simulink model "Level27"  (R2016a)
settings: Solver=VariableStepAuto  StartTime=0.0  StopTime=4/50  MaxStep=1e-6  MinStep=1e-7  RelTol=1e-3
libraries: simulink x26, powerlib x19
settings Model: Creator=satheeshwaran  LastModifiedBy=satheeshwaran

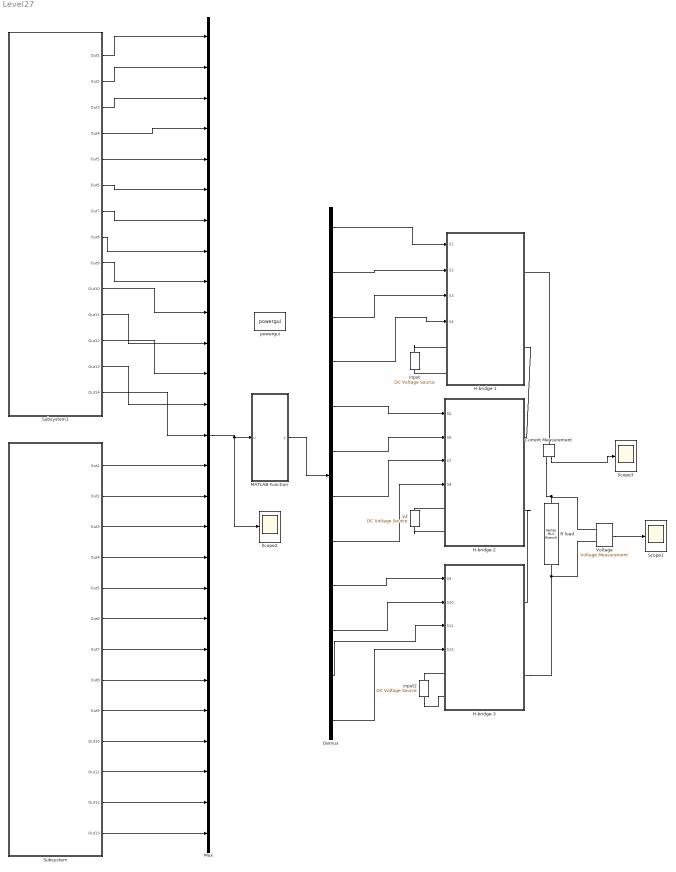
== system Level27 ==
  Current Measurement : powerlib/Measurements/Current Measurement  PhasorSimulation=off  OutputType=Complex  PSBequivalent=0
  Demux : Demux  Outputs=12
  H-bridge-1 : Subsystem
  H-bridge-2 : Subsystem
  H-bridge-3 : Subsystem
  MATLAB Function : MATLAB Function  TreatAsAtomicUnit=on
  Mux : Mux  Inputs=27
  R load : powerlib/Elements/Series RLC Branch  LConnTagsString=__new0  RConnTagsString=__new0  BranchType=R  Resistance=100  Inductance=1e-3  SetiL0=off  InitialCurrent=0  Capacitance=1e-6  Setx0=off  InitialVoltage=0  Measurements=None
  Scope1 : Scope
  Scope2 : Scope
  Scope3 : Scope
  Subsystem : Subsystem
  Subsystem1 : Subsystem
  Voltage : powerlib/Measurements/Voltage Measurement  PhasorSimulation=off  OutputType=Complex  PSBequivalent=0
  input : powerlib/Electrical Sources/DC Voltage Source  Amplitude=100  Measurements=None
  input2 : powerlib/Electrical Sources/DC Voltage Source  Amplitude=900  Measurements=None
  powergui : powerlib/powergui  Priority=1  SimulationMode=Continuous  SolverType=Tustin/Backward Euler (TBE)  SampleTime=50e-6  frequency=60  SPID=off  DisableSnubberDevices=off  DisableRonSwitches=off  DisableVfSwitches=off  SwTol=0  DisplayEquations=off  Interpol=off  ExternalGateDelay=off  methode=off  Ts=10  FunctionMessages=off  echomessages=off  HookPort=off  EnableUseOfTLC=off  x0status=blocks  frequencyindice=0  Pbase=100e6  ErrMax=1e-4  Iterations=50  UnitsV=kV  UnitsW=MW  buscounter=0  RestoreLinks=warning  ResistiveCurrentMeasurement=off  Frange=[0:2:500]  Ylog=off  Xlog=on  ShowGrid=off  save=off  variable=ZData  structure=vload  ZoomFFT=off  StartTime=0.04  cycles=1  DisplayStyle=1  fundamental=50  FreqAxis=off  MaxFrequency=20000  frequencyindicesteady=1  RmsSteady=1  display=off
  v2 : powerlib/Electrical Sources/DC Voltage Source  Amplitude=300  Measurements=None
  wires:
  Voltage/1 -> Scope1/1
  Demux/1 -> H-bridge-1/1(S1)
  Demux/2 -> H-bridge-1/2(S2)
  Demux/5 -> H-bridge-2/1(S5)
  Demux/6 -> H-bridge-2/2(S6)
  Demux/7 -> H-bridge-2/3(S7)
  Demux/9 -> H-bridge-3/1(S9)
  Demux/12 -> H-bridge-3/4(S12)
  Demux/11 -> H-bridge-3/3(S11)
  Demux/10 -> H-bridge-3/2(S10)
  Mux/1 -> Scope2/1, MATLAB Function/1(u)
  MATLAB Function/1(y) -> Demux/1
  Demux/3 -> H-bridge-1/3(S3)
  Demux/4 -> H-bridge-1/4(S4)
  Subsystem1/1(Out1) -> Mux/1
  Subsystem1/2(Out2) -> Mux/2
  Subsystem1/3(Out3) -> Mux/3
  Subsystem1/4(Out4) -> Mux/4
  Subsystem1/5(Out5) -> Mux/5
  Subsystem1/6(Out6) -> Mux/6
  Subsystem1/7(Out7) -> Mux/7
  Subsystem1/8(Out8) -> Mux/8
  Subsystem1/9(Out9) -> Mux/9
  Subsystem1/10(Out10) -> Mux/10
  Subsystem1/11(Out11) -> Mux/11
  Subsystem1/12(Out12) -> Mux/12
  Subsystem1/13(Out13) -> Mux/13
  Subsystem1/14(Out14) -> Mux/14
  Subsystem/1(Out1) -> Mux/15
  Subsystem/2(Out2) -> Mux/16
  Subsystem/3(Out3) -> Mux/17
  Subsystem/4(Out4) -> Mux/18
  Subsystem/5(Out5) -> Mux/19
  Subsystem/6(Out6) -> Mux/20
  Subsystem/7(Out7) -> Mux/21
  Subsystem/8(Out8) -> Mux/22
  Subsystem/9(Out9) -> Mux/23
  Subsystem/10(Out10) -> Mux/24
  Subsystem/11(Out11) -> Mux/25
  Subsystem/12(Out12) -> Mux/26
  Subsystem/13(Out13) -> Mux/27
  Demux/8 -> H-bridge-2/4(S8)
  Current Measurement/1 -> Scope3/1
  connections:
  Voltage/LConn2 -- H-bridge-3/RConn2 -- R load/RConn1
  input2/RConn1 -- H-bridge-3/LConn1
  input2/LConn1 -- H-bridge-3/LConn2
  H-bridge-2/RConn2 -- H-bridge-3/RConn1
  Voltage/LConn1 -- Current Measurement/RConn1 -- R load/LConn1
  H-bridge-1/RConn2 -- H-bridge-2/RConn1
  H-bridge-2/LConn1 -- v2/RConn1
  H-bridge-1/LConn2 -- input/LConn1
  v2/LConn1 -- H-bridge-2/LConn2
  input/RConn1 -- H-bridge-1/LConn1
  Current Measurement/LConn1 -- H-bridge-1/RConn1

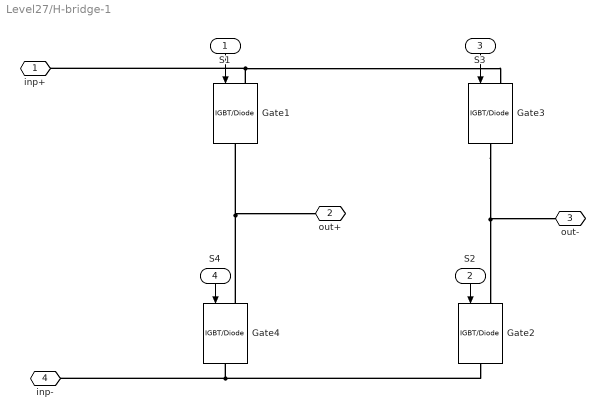
== system Level27/H-bridge-1 ==
  S1 : Inport
  S2 : Inport  Port=2
  S3 : Inport  Port=3
  S4 : Inport  Port=4
  Gate{1..4} (4 alike) : powerlib/Power Electronics/IGBT//Diode  Ron=1e-3  Rs=1e5  Cs=inf  Measurements=off
  inp+ : PMIOPort  Port=1  Side=Left
  out+ : PMIOPort  Port=2  Side=Right
  out- : PMIOPort  Port=3  Side=Right
  inp- : PMIOPort  Port=4  Side=Left
  wires:
  S1/1 -> Gate1/1
  S4/1 -> Gate4/1
  S2/1 -> Gate2/1
  S3/1 -> Gate3/1
  connections:
  Gate2/RConn1 -- inp-/RConn1 -- Gate4/RConn1
  Gate3/RConn1 -- out-/RConn1 -- Gate2/LConn1
  Gate4/LConn1 -- out+/RConn1 -- Gate1/RConn1
  Gate1/LConn1 -- inp+/RConn1 -- Gate3/LConn1

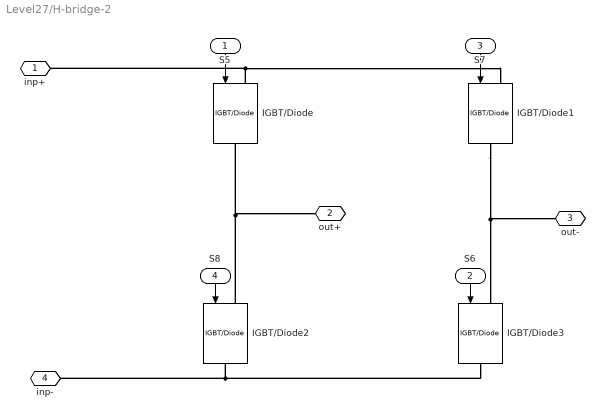
== system Level27/H-bridge-2 ==
  S5 : Inport
  S6 : Inport  Port=2
  S7 : Inport  Port=3
  S8 : Inport  Port=4
  IGBT/Diode{,1..3} (4 alike) : powerlib/Power Electronics/IGBT//Diode  Ron=1e-3  Rs=1e5  Cs=inf  Measurements=off
  inp+ : PMIOPort  Port=1  Side=Left
  out+ : PMIOPort  Port=2  Side=Right
  out- : PMIOPort  Port=3  Side=Right
  inp- : PMIOPort  Port=4  Side=Left
  wires:
  S5/1 -> IGBT/Diode/1
  S8/1 -> IGBT/Diode2/1
  S6/1 -> IGBT/Diode3/1
  S7/1 -> IGBT/Diode1/1
  connections:
  IGBT/Diode3/RConn1 -- inp-/RConn1 -- IGBT/Diode2/RConn1
  IGBT/Diode1/RConn1 -- out-/RConn1 -- IGBT/Diode3/LConn1
  IGBT/Diode2/LConn1 -- out+/RConn1 -- IGBT/Diode/RConn1
  IGBT/Diode/LConn1 -- inp+/RConn1 -- IGBT/Diode1/LConn1

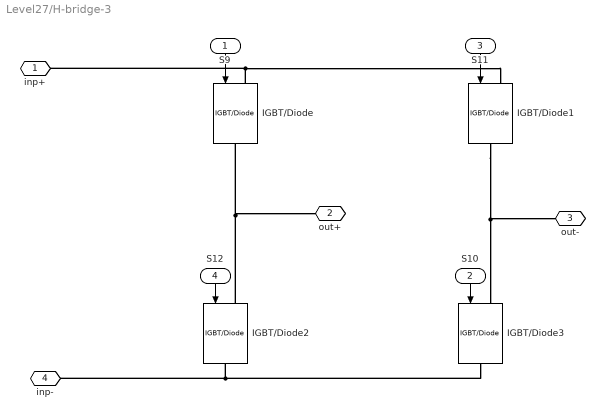
== system Level27/H-bridge-3 ==
  S9 : Inport
  S10 : Inport  Port=2
  S11 : Inport  Port=3
  S12 : Inport  Port=4
  IGBT/Diode{,1..3} (4 alike) : powerlib/Power Electronics/IGBT//Diode  Ron=1e-3  Rs=1e5  Cs=inf  Measurements=off
  inp+ : PMIOPort  Port=1  Side=Left
  out+ : PMIOPort  Port=2  Side=Right
  out- : PMIOPort  Port=3  Side=Right
  inp- : PMIOPort  Port=4  Side=Left
  wires:
  S9/1 -> IGBT/Diode/1
  S12/1 -> IGBT/Diode2/1
  S10/1 -> IGBT/Diode3/1
  S11/1 -> IGBT/Diode1/1
  connections:
  IGBT/Diode3/RConn1 -- inp-/RConn1 -- IGBT/Diode2/RConn1
  IGBT/Diode1/RConn1 -- out-/RConn1 -- IGBT/Diode3/LConn1
  IGBT/Diode2/LConn1 -- out+/RConn1 -- IGBT/Diode/RConn1
  IGBT/Diode/LConn1 -- inp+/RConn1 -- IGBT/Diode1/LConn1

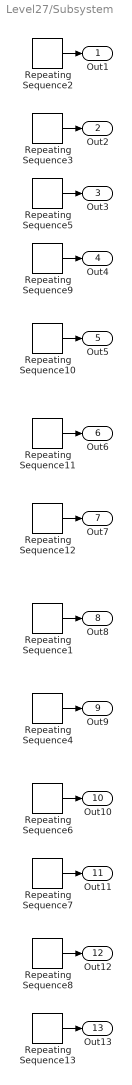
== system Level27/Subsystem ==
  Repeating Sequence1 : simulink/Sources/Repeating Sequence  rep_seq_t=[0 1/20000 1/10000]  rep_seq_y=[-7 -8 -7]
  Repeating Sequence10 : simulink/Sources/Repeating Sequence  rep_seq_t=[0 1/20000 1/10000]  rep_seq_y=[-4 -5 -4]
  Repeating Sequence11 : simulink/Sources/Repeating Sequence  rep_seq_t=[0 1/20000 1/10000]  rep_seq_y=[-5 -6 -5]
  Repeating Sequence12 : simulink/Sources/Repeating Sequence  rep_seq_t=[0 1/20000 1/10000]  rep_seq_y=[-6 -7 -6]
  Repeating Sequence13 : simulink/Sources/Repeating Sequence  rep_seq_t=[0 1/20000 1/10000]  rep_seq_y=[-12 -13 -12]
  Repeating Sequence2 : simulink/Sources/Repeating Sequence  rep_seq_t=[0 1/20000 1/10000]  rep_seq_y=[0 -1 0]
  Repeating Sequence3 : simulink/Sources/Repeating Sequence  rep_seq_t=[0 1/20000 1/10000]  rep_seq_y=[-1 -2 -1]
  Repeating Sequence4 : simulink/Sources/Repeating Sequence  rep_seq_t=[0 1/20000 1/10000]  rep_seq_y=[-8 -9 -8]
  Repeating Sequence5 : simulink/Sources/Repeating Sequence  rep_seq_t=[0 1/20000 1/10000]  rep_seq_y=[-2 -3 -2]
  Repeating Sequence6 : simulink/Sources/Repeating Sequence  rep_seq_t=[0 1/20000 1/10000]  rep_seq_y=[-9 -10 -9]
  Repeating Sequence7 : simulink/Sources/Repeating Sequence  rep_seq_t=[0 1/20000 1/10000]  rep_seq_y=[-10 -11 -10]
  Repeating Sequence8 : simulink/Sources/Repeating Sequence  rep_seq_t=[0 1/20000 1/10000]  rep_seq_y=[-11 -12 -11]
  Repeating Sequence9 : simulink/Sources/Repeating Sequence  rep_seq_t=[0 1/20000 1/10000]  rep_seq_y=[-3 -4 -3]
  Out1 : Outport
  Out2 : Outport  Port=2
  Out3 : Outport  Port=3
  Out4 : Outport  Port=4
  Out5 : Outport  Port=5
  Out6 : Outport  Port=6
  Out7 : Outport  Port=7
  Out8 : Outport  Port=8
  Out9 : Outport  Port=9
  Out10 : Outport  Port=10
  Out11 : Outport  Port=11
  Out12 : Outport  Port=12
  Out13 : Outport  Port=13
  wires:
  Repeating Sequence9/1 -> Out4/1
  Repeating Sequence12/1 -> Out7/1
  Repeating Sequence3/1 -> Out2/1
  Repeating Sequence5/1 -> Out3/1
  Repeating Sequence2/1 -> Out1/1
  Repeating Sequence11/1 -> Out6/1
  Repeating Sequence8/1 -> Out12/1
  Repeating Sequence1/1 -> Out8/1
  Repeating Sequence10/1 -> Out5/1
  Repeating Sequence4/1 -> Out9/1
  Repeating Sequence6/1 -> Out10/1
  Repeating Sequence7/1 -> Out11/1
  Repeating Sequence13/1 -> Out13/1

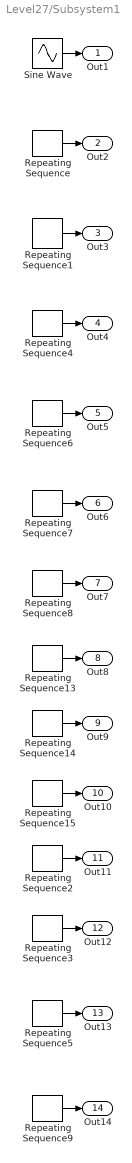
== system Level27/Subsystem1 ==
  Repeating Sequence : simulink/Sources/Repeating Sequence  rep_seq_t=[0 1/20000 1/10000]  rep_seq_y=[0 1 0]
  Repeating Sequence1 : simulink/Sources/Repeating Sequence  rep_seq_t=[0 1/20000 1/10000]  rep_seq_y=[1 2 1]
  Repeating Sequence13 : simulink/Sources/Repeating Sequence  rep_seq_t=[0 1/20000 1/10000]  rep_seq_y=[6 7 6]
  Repeating Sequence14 : simulink/Sources/Repeating Sequence  rep_seq_t=[0 1/20000 1/10000]  rep_seq_y=[7 8 7]
  Repeating Sequence15 : simulink/Sources/Repeating Sequence  rep_seq_t=[0 1/20000 1/10000]  rep_seq_y=[8 9 8]
  Repeating Sequence2 : simulink/Sources/Repeating Sequence  rep_seq_t=[0 1/20000 1/10000]  rep_seq_y=[9 10 9]
  Repeating Sequence3 : simulink/Sources/Repeating Sequence  rep_seq_t=[0 1/20000 1/10000]  rep_seq_y=[10 11 10]
  Repeating Sequence4 : simulink/Sources/Repeating Sequence  rep_seq_t=[0 1/20000 1/10000]  rep_seq_y=[2 3 2]
  Repeating Sequence5 : simulink/Sources/Repeating Sequence  rep_seq_t=[0 1/20000 1/10000]  rep_seq_y=[11 12 11]
  Repeating Sequence6 : simulink/Sources/Repeating Sequence  rep_seq_t=[0 1/20000 1/10000]  rep_seq_y=[3 4 3]
  Repeating Sequence7 : simulink/Sources/Repeating Sequence  rep_seq_t=[0 1/20000 1/10000]  rep_seq_y=[4 5 4]
  Repeating Sequence8 : simulink/Sources/Repeating Sequence  rep_seq_t=[0 1/20000 1/10000]  rep_seq_y=[5 6 5]
  Repeating Sequence9 : simulink/Sources/Repeating Sequence  rep_seq_t=[0 1/20000 1/10000]  rep_seq_y=[12 13 12]
  Sine Wave : Sin  Amplitude=13  Frequency=2*pi*50  SampleTime=0
  Out1 : Outport
  Out2 : Outport  Port=2
  Out3 : Outport  Port=3
  Out4 : Outport  Port=4
  Out5 : Outport  Port=5
  Out6 : Outport  Port=6
  Out7 : Outport  Port=7
  Out8 : Outport  Port=8
  Out9 : Outport  Port=9
  Out10 : Outport  Port=10
  Out11 : Outport  Port=11
  Out12 : Outport  Port=12
  Out13 : Outport  Port=13
  Out14 : Outport  Port=14
  wires:
  Repeating Sequence7/1 -> Out6/1
  Repeating Sequence6/1 -> Out5/1
  Repeating Sequence4/1 -> Out4/1
  Sine Wave/1 -> Out1/1
  Repeating Sequence1/1 -> Out3/1
  Repeating Sequence13/1 -> Out8/1
  Repeating Sequence/1 -> Out2/1
  Repeating Sequence14/1 -> Out9/1
  Repeating Sequence3/1 -> Out12/1
  Repeating Sequence9/1 -> Out14/1
  Repeating Sequence2/1 -> Out11/1
  Repeating Sequence5/1 -> Out13/1
  Repeating Sequence15/1 -> Out10/1
  Repeating Sequence8/1 -> Out7/1

== matlab function Level27/MATLAB Function ==
  data: u input; y output
function y = fcn(u)

sine = u(1);
%Variables  of + carriers
c1 = u(2);
c2 = u(3);
c3 = u(4);
c4 = u(5);
c5 = u(6);
c6 = u(7);
c7 = u(8);
c8 = u(9);
c9 = u(10);
c10 = u(11);
c11= u(12);
c12= u(13);
c13 = u(14);

%Variables  of - carriers
n1 = u(15);
n2 = u(16);
n3 = u(17);
n4 = u(18);
n5 = u(19);
n6 = u(20);
n7 = u(21);
n8 = u(22);
n9 = u(23);
n10 = u(24);
n11 = u(25);
n12 = u(26);
n13 = u(27);

s1 = 0;
s3 = 0;
s5 = 0;
s7 = 0;
s2 = 0;
s4 = 0;
s6 = 0;
s8 = 0;
s9 = 0;
s10 = 0;
s11 = 0;
s12 = 0;
% 0 - 100v
if (sine >= 0 && sine < 1)
    if (sine >= c1)
        s1 = 1;s2=1;s5=1;s7=1;s9=1;s11=1;
    else
        s1 = 1;s3=1;s5=1;s7=1;s9=1;s11=1;
    end
end
%100 - 200
if (sine >= 1 && sine < 2)
    if (sine >= c2)
        s3 = 1;s4=1;s5=1;s6=1;s9=1;s11=1;
    else
         s1 = 1;s2=1;s5=1;s7=1;s9=1;s11=1;
    end
end
%200 - 300
if (sine >= 2 && sine < 3)
    if (sine >= c3)
        s1 = 1;s3=1;s5=1;s6=1;s9=1;s11=1;
    else
        s3 = 1;s4=1;s5=1;s6=1;s9=1;s11=1;
    end
end
%300 - 400
if (sine >= 3 && sine < 4)
    if (sine >= c4)
        s1 = 1;s2=1;s5=1;s6=1;s9=1;s11=1;
    else
         s1 = 1;s3=1;s5=1;s6=1;s9=1;s11=1;
    end
end
%400 - 500
if (sine >= 4 && sine < 5)
    if (sine >= c5)
        s3 = 1;s4=1;s8=1;s7=1;s10=1;s9=1;
    else
        s1 = 1;s2=1;s5=1;s6=1;s9=1;s11=1;
    end
end
%500 - 600
if (sine >= 5 && sine < 6)
    if (sine >= c6)
        s1 = 1;s3=1;s7=1;s8=1;s9=1;s10=1;
    else
       s3 = 1;s4=1;s8=1;s7=1;s10=1;s9=1;
    end
end
%600 - 700
if (sine >= 6 && sine < 7)
    if (sine >= c7)
        s1 = 1;s2=1;s7=1;s8=1;s9=1;s10=1;
    else
        s1 = 1;s3=1;s7=1;s8=1;s9=1;s10=1;
    end
end
%700 - 800
if (sine >= 7 && sine < 8)
    if (sine >= c8)
        s3 = 1;s4=1;s5=1;s7=1;s9=1;s10=1;
    else
        s1 = 1;s2=1;s7=1;s8=1;s9=1;s10=1;
    end
end
%800 - 900
if (sine >= 8 && sine < 9)
    if (sine >= c9)
        s1 = 1;s3=1;s5=1;s7=1;s9=1;s10=1;
    else
        s3 = 1;s4=1;s5=1;s7=1;s9=1;s10=1;
    end
end
%900 - 1000
if (sine >= 9 && sine < 10)
    if (sine >= c10)
        s1 = 1;s2=1;s5=1;s7=1;s9=1;s10=1;
    else
        s1 = 1;s3=1;s5=1;s7=1;s9=1;s10=1;
    end
end
%1000 - 1100
if (sine >= 10 && sine < 11)
    if (sine >= c11)
        s3 = 1;s4=1;s5=1;s6=1;s9=1;s10=1;
    else
        s1 = 1;s2=1;s5=1;s7=1;s9=1;s10=1;
    end
end
%1100 - 1200
if (sine >= 11 && sine < 12)
    if (sine >= c12)
        s1 = 1;s3=1;s5=1;s6=1;s9=1;s10=1;
    else
        s3 = 1;s4=1;s5=1;s6=1;s9=1;s10=1;
    end
end
%1200 - 1300
if (sine >= 12 && sine <= 13)
    if (sine >= c13)
        s1 = 1;s2=1;s5=1;s6=1;s9=1;s10=1;
    else
        s1 = 1;s3=1;s5=1;s6=1;s9=1;s10=1;
    end
end
%0 : -100
if (sine < 0 && sine >= -1)
    if (sine <= n1)
        s3 = 1;s4=1;s5=1;s7=1;s9=1;s11=1;
    else
        s1 = 1;s3=1;s5=1;s7=1;s9=1;s11=1;
    end
end
% -100 : -200
if (sine < -1 && sine >= -2)
    if (sine <= n2)
        s1= 1;s2=1;s8=1;s7=1;s9=1;s11=1;
    else
         s3 = 1;s4=1;s5=1;s7=1;s9=1;s11=1;
    end
end
% -200 : -300
if (sine < -2 && sine >= -3)
    if (sine <= n3)
        s1= 1;s3=1;s8=1;s7=1;s9=1;s11=1;
    else
          s1= 1;s2=1;s8=1;s7=1;s9=1;s11=1;
    end
end
% -300 : -400
if (sine < -3 && sine >= -4)
    if (sine <= n4)
        s4 = 1;s3=1;s8=1;s7=1;s9=1;s11=1;
    else
        s1= 1;s3=1;s8=1;s7=1;s9=1;s11=1;
    end
end
% -400 : -500
if (sine < -4 && sine >= -5)
    if (sine <= n5)
        s1 = 1;s2=1;s5=1;s6=1;s12=1;s11=1;
    else
        s4 = 1;s3=1;s8=1;s7=1;s9=1;s11=1;
    end
end
% -500 : -600
if (sine < -5 && sine > -6)
    if (sine <= n6)
        s1 = 1;s3=1;s5=1;s6=1;s12=1;s11=1;
    else
        s1 = 1;s2=1;s5=1;s6=1;s12=1;s11=1;
    end
end
% -600 : -700
if (sine < -6 && sine >= -7)
    if (sine <= n7)
        s4 = 1;s3=1;s5=1;s6=1;s12=1;s11=1;
    else
        s1 = 1;s3=1;s5=1;s6=1;s12=1;s11=1;
    end
end
%-700 : -800
if (sine < -7 && sine >= -8)
    if (sine <= n8)
        s1 = 1;s2=1;s5=1;s7=1;s12=1;s11=1;
    else
        s4 = 1;s3=1;s5=1;s6=1;s12=1;s11=1;
    end
end
% -800 : -900
if (sine < -8 && sine >= -9)
    if (sine <= n9)
        s1= 1;s3=1;s5=1;s7=1;s12=1;s11=1;
    else
        s1 = 1;s2=1;s5=1;s7=1;s12=1;s11=1;
    end
end
% -900 : -1000
if (sine < -9  &&  sine >= -10)
    if (sine <= n10)
        s3= 1;s4=1;s5=1;s7=1;s12=1;s11=1;
    else
          s1= 1;s3=1;s5=1;s7=1;s12=1;s11=1;
    end
end
% -1000 : -1100
if (sine < -10 && sine >= -11)
    if (sine <= n11)
        s1 = 1;s2=1;s8=1;s7=1;s12=1;s11=1;
    else
        s3= 1;s4=1;s5=1;s7=1;s12=1;s11=1;
    end
end
% -1100 : -1200
if (sine < -11 && sine >= -12)
    if (sine <= n12)
        s1 = 1;s3=1;s8=1;s7=1;s12=1;s11=1;
    else
         s1 = 1;s2=1;s8=1;s7=1;s12=1;s11=1;
    end
end
% -1200 : -1300
if (sine < -12 && sine >= -13)
    if (sine <= n13)
        s4 = 1;s3=1;s7=1;s8=1;s12=1;s11=1;
    else
        s1 = 1;s3=1;s8=1;s7=1;s12=1;s11=1;
    end
end

y = [s1; s2; s3; s4; s5; s6; s7; s8; s9; s10; s11; s12];
